simulink model "streaming_icecast"  (R2015a)
settings: Solver=ode45  StartTime=0.0  StopTime=10000  RelTol=1e-3
settings Model: Creator=windor  LastModifiedBy=windor

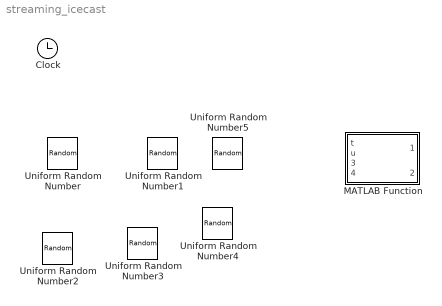
== system streaming_icecast ==
  Clock : Clock
  MATLAB Function : MATLAB Function  TreatAsAtomicUnit=on
  Uniform Random Number{,1..5} (6 alike) : UniformRandomNumber  SampleTime=0.1

== matlab function streaming_icecast/MATLAB Function ==
  data: t input; u input; nueva_llegada output; lambda input; tiempo_ultima_llegada input; tiempo_prox_llegada output
function [nueva_llegada, tiempo_prox_llegada] = generador_llegadas(t, u, lambda, tiempo_ultima_llegada)
% Genera eventos de llegada según proceso de Poisson

persistent tiempo_proxima;

if isempty(tiempo_proxima)
    tiempo_proxima = 0;
end

nueva_llegada = 0;

% Verificar si es momento de nueva llegada
if t >= tiempo_proxima
    nueva_llegada = 1;
    % Generar próximo tiempo entre llegadas
    tiempo_entre = -log(u) / lambda;
    tiempo_proxima = t + tiempo_entre;
end

tiempo_prox_llegada = tiempo_proxima;
